simulink model "Fuzzy_Logic_controller"  (R2023a)
settings: Solver=ode23t  StartTime=0.0  StopTime=1.5  MaxStep=0.1  RelTol=1e-4
undefined symbols (not defined in the file): Fuzzy_Logic_parameters, Linear_part
libraries: fuzblock x1
settings Model: Creator=ПК  LastModifiedBy=ПК

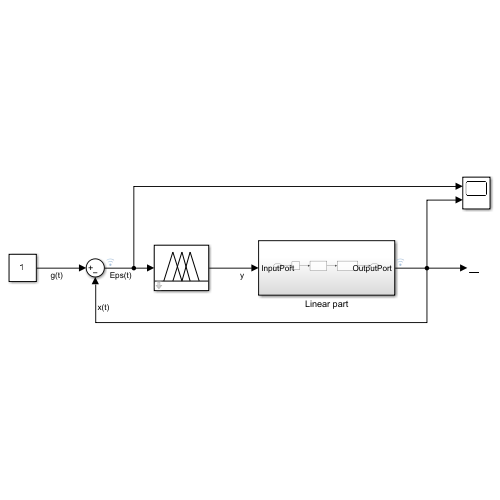
[thumbnail: Simulink's stored preview of the top-level diagram]
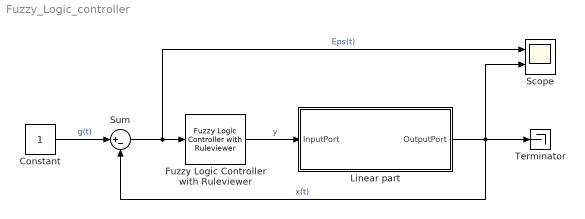
== system Fuzzy_Logic_controller ==
  Constant : Constant
  Fuzzy Logic Controller with Ruleviewer : fuzblock/Fuzzy Logic  Controller  with Ruleviewer  fismatrix=Fuzzy_Logic_settings  Ts=Fuzzy_Logic_parameters.Ts
  Linear part : Subsystem
  Scope : Scope  NumInputPorts=2
  Sum : Sum  Inputs=|+-
  Terminator : Terminator
  wires:
  Constant/1 -> Sum/1  "g(t)"
  Linear part/1(OutputPort) -> Scope/2, Terminator/1, Sum/2  "x(t)"
  Fuzzy Logic Controller with Ruleviewer/1 -> Linear part/1(InputPort)  "y"
  Sum/1 -> Fuzzy Logic Controller with Ruleviewer/1, Scope/1  "Eps(t)"

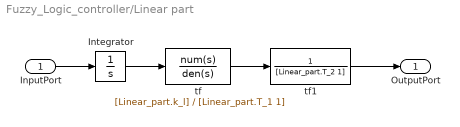
== system Fuzzy_Logic_controller/Linear part ==
  InputPort : Inport
  Integrator : Integrator
  tf : TransferFcn  Numerator=[Linear_part.k_l]  Denominator=[Linear_part.T_1 1]
  tf1 : TransferFcn  Denominator=[Linear_part.T_2 1]
  OutputPort : Outport
  wires:
  InputPort/1 -> Integrator/1
  Integrator/1 -> tf/1
  tf/1 -> tf1/1
  tf1/1 -> OutputPort/1
